simulink model "Main"  (Simulink 6.6)
settings: Solver=FixedStepDiscrete  StartTime=0.0  StopTime=Inf  FixedStep=0.001  RelTol=1e-3
undefined symbols (not defined in the file): ecan1_init, ecan1_receive_matlab, ecan1_transmit_matlab, u1, y1
libraries: simulink x83, dsPICdrivers x6
(part 2 of 2)

== matlab function Configure ECAN 1/Subsystem4/Embedded MATLAB Function ==
  settings: updateMethod=DISCRETE  sampleTime=Inf
  data: sel1 output inherited; sel2 output inherited; filters input inherited; filter_masks input inherited
function [sel1,sel2] = buildMaskSelReg(filters, filter_masks)

sel1 = uint16(0);
sel2 = uint16(0);
for k = 1:size(filters,1);
    filter = filters(k)+1;
    if filter < 9 % 9 because of 1-indexing in MATLAB
        sel1 = bitor(sel1, bitshift(filter_masks(filter),2*k));
    else
        sel2 = bitor(sel2, bitshift(filter_masks(filter),2*(k-8)));
    end
end
